simulink model "closedLoop_SpO2H"  (Simulink 10.0)
settings: Solver=ode23t  StartTime=0.0  StopTime=2000  FixedStep=0.01  RelTol=1e-6  AbsTol=1e-9
model workspace: external: MAT-File parL3.mat (data not in the file)
values from neighbouring files (symbols this model uses):
  a0 = parRp(3)    [calcAuxVars.m]    (also in parL.mat = [1.15338450687 1.39375935389 0.940877756773 0.999834385293 0; parL0.mat = [1.15338450687 1.39375935389 0.940877756773 0.999834385293 0; parL1.mat = [1.15338450687 1.39375935389 0.940877756773 0.999834385293 0; parL2.mat = [1.15338450687 1.39375935389 0.940877756773 0.999834385293 0)
  a1 = parRp(4)    [calcAuxVars.m]    (also in parL.mat = [0.343538892932 0.21152716103 0.0176956627984 0.500319126811; parL0.mat = [0.343538892932 0.21152716103 0.0176956627984 0.500319126811; parL1.mat = [0.343538892932 0.21152716103 0.0176956627984 0.500319126811; parL2.mat = [0.343538892932 0.21152716103 0.0176956627984 0.500319126811)
  a_p0 = 0.5    [parL.mat]    (also in parL0.mat; parL1.mat; parL2.mat; parL3.mat)
  b_p0 = 1.1    [parL.mat]    (also in parL0.mat; parL1.mat; parL2.mat; parL3.mat)
  c0 = parRp(5)    [calcAuxVars.m]    (also in parL.mat = [2.87886478699 3.35726152565 2.07888198195 3.00150379853 2.7; parL0.mat = [2.87886478699 3.35726152565 2.07888198195 3.00150379853 2.7; parL1.mat = [2.87886478699 3.35726152565 2.07888198195 3.00150379853 2.7; parL2.mat = [2.87886478699 3.35726152565 2.07888198195 3.00150379853 2.7)
  In_T = [4.28 3.84 4.92 31.48 4.84 4.16 4.04 6.28 22.04 4.52 4.2 4.2 ... (112 elements, 1x112)]    [parL.mat]    (also in parL0.mat; parL1.mat; parL2.mat; parL3.mat)
  InInspirT = [3.74988154254 3.29053790944 2.30955999915 3.3968770932 3.63249544085 3.4615806603 3.39373309529 2.87032279982 2.30291149597 3.50313332581 3.84662991695 3.66498954271 ... (112 elements, 112x1)]    [parL.mat]    (also in parL0.mat; parL1.mat; parL2.mat; parL3.mat)
  Ki = 0.0002    [parL.mat]    (also in parL0.mat; parL1.mat; parL2.mat = 0.002; parL3.mat = 0.002)
  Kp = 0.01    [parL.mat]    (also in parL0.mat = 0.04; parL1.mat = 0.04; parL2.mat = 0.4; parL3.mat = 0.4)
  LRI = 7.5    [parL.mat]    (also in parL0.mat; parL1.mat; parL2.mat = 6.5; parL3.mat = 6.5)
  Rp_adjust = 1    [parL.mat]    (also in parL0.mat; parL1.mat; parL2.mat; parL3.mat)
  SAo_set = 96    [parL2.mat]    (also in parL3.mat)
  taf = parRp(1)    [calcAuxVars.m]    (also in parL.mat = [0.808561437671 0.693291047527 0.236392042426 0.798691385589; parL0.mat = [0.808561437671 0.693291047527 0.236392042426 0.798691385589; parL1.mat = [0.808561437671 0.693291047527 0.236392042426 0.798691385589; parL2.mat = [0.808561437671 0.693291047527 0.236392042426 0.798691385589)
  tbf = parRp(2)+parRp(1)    [calcAuxVars.m]    (also in parL.mat = [1.94132010487 1.59724686191 1.07316795672 1.59818570761 1.9; parL0.mat = [1.94132010487 1.59724686191 1.07316795672 1.59818570761 1.9; parL1.mat = [1.94132010487 1.59724686191 1.07316795672 1.59818570761 1.9; parL2.mat = [1.94132010487 1.59724686191 1.07316795672 1.59818570761 1.9)
  x0 = xi(end,:)    [fitLung_slp60m1.m]    (also in fitLung_slp67xm.m; fitSpO2_slp60m1.m; fitSpO2_slp67xm.m; initialVariables.m = [x1;x2;x3;x4;x5;x6;x7;x8;x9;x10;x11;x12])
libraries: dspsigops x8, simulink x1
settings Model: Creator=ceic208  LastModifiedBy=wai484  SimulationMode=accelerator  PauseTimes=12.2274
settings Model: LogicAnalyzerGraphicalSettings=|
  | {
  |   "cursors" : {
  |     "activeCursor" : 0,
  |     "lockedCursors" : [
  | 
  |     ],
  |     "startingCursor" : 0,
  |     "times" : [
  |       0
  |     ]
  |   },
  |   "global" : {
  |   },
  |   "panels" : [
  |     {
  |       "height" : 100,
  |       "startingTrace" : 0,
  |       "traces" : [
  |         {
  |           "signalId" : "c403b30c-f251-48ef-8f45-5741095cfd99",
  |           "type" : "wave"
  |         },
  |         {
  |           "signalId" : "18fa4ba5-052e-4074-9df1-028c4f90615a",
  |           "type" : "wave"
  |         },
  |         {
  |           "signalId" : "c514b470-b808-4634-b1ae-82d406deb028",
  |           "type" : "wave"
  |         },
  |         {
  |           "signalId" : "1a470e6e-5724-4372-8d16-b9d493f2bf0a",
  |           "type" : "wave"
  |         }
  |       ],
  |       "yOffset" : 0
  |     }
  |   ],
  |   "timeAxis" : {
  |     "pixelsPerSecond" : 0.4395
  |   },
  |   "trigger" : {
  |     "enabled" : false,
  |     "mode" : "once",
  |     "samples" : 200,
  |     "signals" : {
  |     },
  |     "stages" : [
  |       {
  |         "conditions" : [
  | 
  |         ],
  |         "operator" : "AND"
  |       }
  |     ]
  |   }
  | }
settings DataIOCC: SignalLogging=off  DSMLogging=off
settings OptimizationCC: LifeSpan=auto
settings DebuggingCC: UnderspecifiedInitializationDetection=Simplified  MergeDetectMultiDrivingBlocksExec=error  SFUnexpectedBacktrackingDiag=error  SFNoUnconditionalDefaultTransitionDiag=error  SFExecutionAtInitializationDiag=warning
settings HardwareCC: ProdBitPerPointer=64  ProdBitPerSizeT=64  ProdBitPerPtrDiffT=64  ProdLargestAtomicFloat=Float  ProdIntDivRoundTo=Zero  ProdEndianess=LittleEndian  ProdWordSize=64  ProdHWDeviceType=Intel->x86-64 (Windows64)
settings ModelReferenceCC: PropagateSignalLabelsOutOfModel=on
settings GRTTargetCC: TargetLangStandard=C99 (ISO)  CombineOutputUpdateFcns=on  GRTInterface=off
settings ConfigComp: CovMetricSettings=dwe  CovSaveCumulativeToWorkspaceVar=off  CovSaveSingleToWorkspaceVar=off

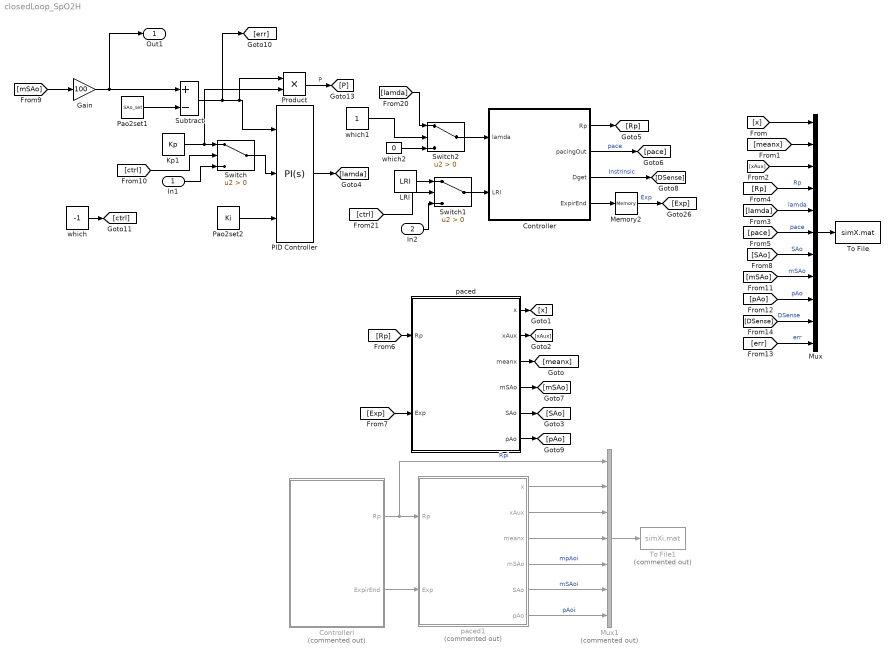
== system closedLoop_SpO2H ==
  In1 : Inport
  In2 : Inport  Port=2
  Controller : Stateflow chart  TreatAsAtomicUnit=on
  Controlleri : Stateflow chart  Commented=on  TreatAsAtomicUnit=on
  Gain : Gain  Gain=100
  Kp1 : Constant  Value=Kp  VectorParams1D=off
  LRI : Constant  Value=LRI  VectorParams1D=off
  Memory2 : Memory
  Mux : Mux  Inputs=11
  Mux1 : Mux  Commented=on  Inputs=7
  PID Controller : simulink/Continuous/PID Controller  Controller=PI  Form=Parallel  TimeDomain=Continuous-time  SampleTime=-1  IntegratorMethod=Forward Euler  FilterMethod=Forward Euler  ControllerParametersSource=external  P=Kp  I=Ki  D=0.00000000001  UseFilter=on  N=100  TunerSelectOption=Transfer Function Based (PID Tuner App)  InitialConditionSource=internal  InitialConditionForIntegrator=0  InitialConditionForFilter=0  DifferentiatorICPrevScaledInput=0  ExternalReset=none  TrackingMode=off  Kt=1  LimitOutput=on  UpperSaturationLimit=0.5  LowerSaturationLimit=-1.5  LinearizeAsGain=on  AntiWindupMode=none  Kb=1  POutMin=[]  POutMax=[]  IOutMin=[]  IOutMax=[]  DOutMin=[]  DOutMax=[]  NOutMin=[]  NOutMax=[]  SumOutMin=[]  SumOutMax=[]  SaturationOutMin=[]  SaturationOutMax=[]  PParamMin=[]  PParamMax=[]  IParamMin=[]  IParamMax=[]  DParamMin=[]  DParamMax=[]  NParamMin=[]  NParamMax=[]  KbParamMin=[]  KbParamMax=[]  KtParamMin=[]  KtParamMax=[]  KbOutMin=[]  KbOutMax=[]  KtOutMin=[]  KtOutMax=[]  IntegratorOutMin=[]  IntegratorOutMax=[]  FilterOutMin=[]  FilterOutMax=[]  SumI1OutMin=[]  SumI1OutMax=[]  SumI2OutMin=[]  SumI2OutMax=[]  SumI3OutMin=[]  SumI3OutMax=[]  SumI4OutMin=[]  SumI4OutMax=[]  SumDOutMin=[]  SumDOutMax=[]  DifferentiatorOutMin=[]  DifferentiatorOutMax=[]  FilterDiffOutCoefMin=[]  FilterDiffOutCoefMax=[]  ReciprocalOutMin=[]  ReciprocalOutMax=[]  SumDenOutMin=[]  SumDenOutMax=[]  SumNumOutMin=[]  SumNumOutMax=[]  DivideOutMin=[]  DivideOutMax=[]  IntegratorContinuousStateAttributes=''  IntegratorStateMustResolveToSignalObject=off  IntegratorRTWStateStorageClass=Auto  FilterContinuousStateAttributes=''  FilterStateMustResolveToSignalObject=off  FilterRTWStateStorageClass=Auto  ParallelPVariant=ExternalParameters  IdealPVariant=Disabled  IVariant=ExternalParameters  DVariant=Disabled  IntegratorVariant=Continuous  SatVariant=Enabled  AWVariant=Passthrough  PCopyVariant=Disabled  TRVariant=Disabled  FdbkBlocksVariant=Forward  IdealPFdbkVariant=Disabled  SatFdbkVariant=Disabled  DerivativeFilterVariant=Disabled  NVariant=Disabled  NCopyVariant=Disabled_SignalSpec  FilterICVariant=Disabled  IntegratorICVariant=InternalICs  ExternalResetVariant=Disabled  TRSumVariant=Passthrough  SumFdbkVariant=Disabled  SumVariant=Sum_PI
  Pao2set1 : Constant  Value=SAo_set  VectorParams1D=off
  Pao2set2 : Constant  Value=Ki  VectorParams1D=off
  Product : Product
  Subtract : Sum  Inputs=+-
  Switch : Switch  Criteria=u2 > Threshold
  Switch1 : Switch  Criteria=u2 > Threshold
  Switch2 : Switch  Criteria=u2 > Threshold
  To File : ToFile  Filename=simX.mat  MatrixName=simX
  To File1 : ToFile  Commented=on  Filename=simXi.mat  MatrixName=simXi
  paced : Subsystem
  paced1 : Subsystem  Commented=on
  which : Constant  Value=-1  VectorParams1D=off
  which1 : Constant  VectorParams1D=off
  which2 : Constant  Value=0  VectorParams1D=off
  Out1 : Outport  PortDimensions=1  VectorParamsAs1DForOutWhenUnconnected=off
  wires:
  Pao2set1/1 -> Subtract/2
  Subtract/1 -> [err], Product/1, PID Controller/1
  [x] -> Mux/1
  [meanx] -> Mux/2
  [xAux] -> Mux/3
  [Rp] -> Mux/4  "Rp"
  [lamda] -> Mux/5  "lamda"
  [pace] -> Mux/6  "pace"
  Mux/1 -> To File/1
  Controller/1(Rp) -> [Rp]
  Pao2set2/1 -> PID Controller/3
  PID Controller/1 -> [lamda]
  Controller/2(pacingOut) -> [pace]  "pace"
  Controller/3(Dget) -> [DSense]  "Instrinsic"
  Switch/1 -> PID Controller/2
  Kp1/1 -> Product/2, Switch/1
  In1/1 -> Switch/3
  which/1 -> [ctrl]
  [ctrl] -> Switch/2
  Switch1/1 -> Controller/2(LRI)
  LRI/1 -> Switch1/1
  In2/1 -> Switch1/3
  [ctrl] -> Switch1/2
  Memory2/1 -> [Exp]  "Exp"
  Controller/4(ExpirEnd) -> Memory2/1
  Product/1 -> [P]  "P"
  paced/3(meanx) -> [meanx]
  paced/1(x) -> [x]
  paced/2(xAux) -> [xAux]
  [Rp] -> paced/1(Rp)
  [Exp] -> paced/2(Exp)
  paced/5(SAo) -> [SAo]
  [SAo] -> Mux/7  "SAo"
  [mSAo] -> Mux/8  "mSAo"
  Controlleri/1(Rp) -> paced1/1(Rp), Mux1/1  "Rpi"
  Controlleri/2(ExpirEnd) -> paced1/2(Exp)
  Mux1/1 -> To File1/1
  paced1/1(x) -> Mux1/2
  paced/6(pAo) -> [pAo]
  paced1/2(xAux) -> Mux1/3
  paced1/3(meanx) -> Mux1/4
  paced1/4(mSAo) -> Mux1/5  "mpAoi"
  paced1/5(SAo) -> Mux1/6  "mSAoi"
  paced1/6(pAo) -> Mux1/7  "pAoi"
  [pAo] -> Mux/9  "pAo"
  [err] -> Mux/11  "err"
  [DSense] -> Mux/10  "DSense"
  [mSAo] -> Gain/1
  Gain/1 -> Out1/1, Subtract/1
  Switch2/1 -> Controller/1(lamda)
  [lamda] -> Switch2/1
  which1/1 -> Switch2/2
  which2/1 -> Switch2/3
  paced/4(mSAo) -> [mSAo]

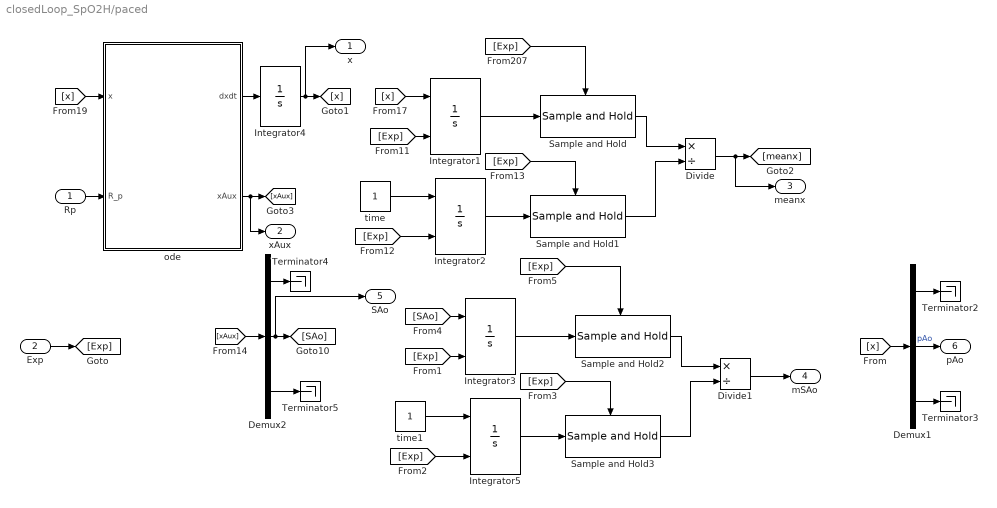
== system closedLoop_SpO2H/paced ==
  Rp : Inport
  Exp : Inport  Port=2
  Demux1 : Demux  Outputs=[6,1,5]
  Demux2 : Demux  Outputs=[13,1,1]
  Divide : Product  Inputs=*/
  Divide1 : Product  Inputs=*/
  Integrator{1..3,5} (4 alike) : Integrator  ExternalReset=either  LimitOutput=on  LowerSaturationLimit=0
  Integrator4 : Integrator  InitialCondition=x0  LimitOutput=on  LowerSaturationLimit=0
  Sample and Hold : dspsigops/Sample and Hold  trig=Either edge  initCond=x0  latchinput=on
  Sample and Hold1 : dspsigops/Sample and Hold  trig=Either edge  initCond=3  latchinput=on
  Sample and Hold2 : dspsigops/Sample and Hold  trig=Either edge  initCond=SAo_set/100*3  latchinput=on
  Sample and Hold3 : dspsigops/Sample and Hold  trig=Either edge  initCond=3  latchinput=on
  Terminator{2..5} (4 alike) : Terminator
  ode : MATLAB Function  TreatAsAtomicUnit=on
  time : Constant  VectorParams1D=off
  time1 : Constant  VectorParams1D=off
  x : Outport  VectorParamsAs1DForOutWhenUnconnected=off
  xAux : Outport  Port=2  VectorParamsAs1DForOutWhenUnconnected=off
  meanx : Outport  Port=3  VectorParamsAs1DForOutWhenUnconnected=off
  mSAo : Outport  Port=4  VectorParamsAs1DForOutWhenUnconnected=off
  SAo : Outport  Port=5  VectorParamsAs1DForOutWhenUnconnected=off
  pAo : Outport  Port=6  VectorParamsAs1DForOutWhenUnconnected=off
  wires:
  Divide/1 -> meanx/1, [meanx]
  time/1 -> Integrator2/1
  Demux2/2 -> SAo/1, [SAo]
  [Exp] -> Sample and Hold1/Trigger
  [Exp] -> Integrator2/2
  Sample and Hold/1 -> Divide/1
  Sample and Hold1/1 -> Divide/2
  [Exp] -> Integrator1/2
  Integrator4/1 -> x/1, [x]
  Integrator2/1 -> Sample and Hold1/1
  Integrator1/1 -> Sample and Hold/1
  [x] -> Integrator1/1
  [x] -> ode/1(x)
  ode/2(xAux) -> xAux/1, [xAux]
  ode/1(dxdt) -> Integrator4/1
  [xAux] -> Demux2/1
  Demux2/1 -> Terminator4/1
  [Exp] -> Sample and Hold/Trigger
  Demux2/3 -> Terminator5/1
  Rp/1 -> ode/2(R_p)
  Exp/1 -> [Exp]
  [x] -> Demux1/1
  Demux1/1 -> Terminator2/1
  Demux1/3 -> Terminator3/1
  Demux1/2 -> pAo/1  "pAo"
  [Exp] -> Sample and Hold2/Trigger
  Divide1/1 -> mSAo/1
  Sample and Hold2/1 -> Divide1/1
  Integrator5/1 -> Sample and Hold3/1
  Sample and Hold3/1 -> Divide1/2
  [Exp] -> Integrator5/2
  Integrator3/1 -> Sample and Hold2/1
  [SAo] -> Integrator3/1
  [Exp] -> Integrator3/2
  [Exp] -> Sample and Hold3/Trigger
  time1/1 -> Integrator5/1

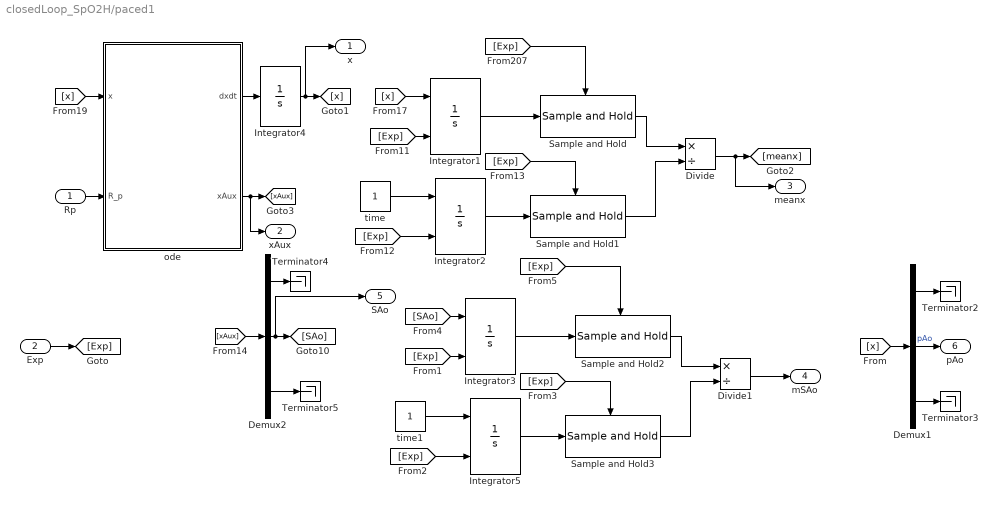
== system closedLoop_SpO2H/paced1 ==
  Rp : Inport
  Exp : Inport  Port=2
  Demux1 : Demux  Outputs=[6,1,5]
  Demux2 : Demux  Outputs=[13,1,1]
  Divide : Product  Inputs=*/
  Divide1 : Product  Inputs=*/
  Integrator{1..3,5} (4 alike) : Integrator  ExternalReset=either  LimitOutput=on  LowerSaturationLimit=0
  Integrator4 : Integrator  InitialCondition=x0  LimitOutput=on  LowerSaturationLimit=0
  Sample and Hold : dspsigops/Sample and Hold  trig=Either edge  initCond=x0  latchinput=on
  Sample and Hold1 : dspsigops/Sample and Hold  trig=Either edge  initCond=3  latchinput=on
  Sample and Hold2 : dspsigops/Sample and Hold  trig=Either edge  initCond=SAo_set/100*3  latchinput=on
  Sample and Hold3 : dspsigops/Sample and Hold  trig=Either edge  initCond=3  latchinput=on
  Terminator{2..5} (4 alike) : Terminator
  ode : MATLAB Function  TreatAsAtomicUnit=on
  time : Constant  VectorParams1D=off
  time1 : Constant  VectorParams1D=off
  x : Outport  VectorParamsAs1DForOutWhenUnconnected=off
  xAux : Outport  Port=2  VectorParamsAs1DForOutWhenUnconnected=off
  meanx : Outport  Port=3  VectorParamsAs1DForOutWhenUnconnected=off
  mSAo : Outport  Port=4  VectorParamsAs1DForOutWhenUnconnected=off
  SAo : Outport  Port=5  VectorParamsAs1DForOutWhenUnconnected=off
  pAo : Outport  Port=6  VectorParamsAs1DForOutWhenUnconnected=off
  wires:
  Divide/1 -> meanx/1, [meanx]
  time/1 -> Integrator2/1
  Demux2/2 -> SAo/1, [SAo]
  [Exp] -> Sample and Hold1/Trigger
  [Exp] -> Integrator2/2
  Sample and Hold/1 -> Divide/1
  Sample and Hold1/1 -> Divide/2
  [Exp] -> Integrator1/2
  Integrator4/1 -> x/1, [x]
  Integrator2/1 -> Sample and Hold1/1
  Integrator1/1 -> Sample and Hold/1
  [x] -> Integrator1/1
  [x] -> ode/1(x)
  ode/2(xAux) -> xAux/1, [xAux]
  ode/1(dxdt) -> Integrator4/1
  [xAux] -> Demux2/1
  Demux2/1 -> Terminator4/1
  [Exp] -> Sample and Hold/Trigger
  Demux2/3 -> Terminator5/1
  Rp/1 -> ode/2(R_p)
  Exp/1 -> [Exp]
  [x] -> Demux1/1
  Demux1/1 -> Terminator2/1
  Demux1/3 -> Terminator3/1
  Demux1/2 -> pAo/1  "pAo"
  [Exp] -> Sample and Hold2/Trigger
  Divide1/1 -> mSAo/1
  Sample and Hold2/1 -> Divide1/1
  Integrator5/1 -> Sample and Hold3/1
  Sample and Hold3/1 -> Divide1/2
  [Exp] -> Integrator5/2
  Integrator3/1 -> Sample and Hold2/1
  [SAo] -> Integrator3/1
  [Exp] -> Integrator3/2
  [Exp] -> Sample and Hold3/Trigger
  time1/1 -> Integrator5/1

== matlab function paced/ode ==
  data: dxdt output double; x input double; xAux output double; R_p input double; parL parameter double
% Calculates derivatives given x & t

function [dxdt,xAux] = odeSystem_LungSim(x,R_p, parL)

P_A = x(1);
f_o = x(2);
f_c = x(3);
f_do = x(4);
f_dc = x(5);
p_Vo = x(6);
p_Ao = x(7);
p_Vc = x(8);
p_Ac = x(9);
z_V = x(10);
z_A = x(11);
x_m=x(12);

[xAux] = calcAuxVarsSim(x,R_p, parL);

P_L = xAux(1);
dP_Ldt = xAux(2);
Q_A = xAux(3);
q = xAux(4);
p_ao = xAux(5);
p_ac = xAux(6);
V_A = xAux(7);
f_o_cos = xAux(8);
f_c_cos = xAux(9);
f_do_cos = xAux(10);
f_dc_cos = xAux(11);
dfpVodpVo = xAux(12);
dfpAodpAo = xAux(13);
S_Ao=xAux(14);
S_Vo=xAux(15);

p_bo = p_Ao; % p_b = partial pressure in pulmonary capillaries which does the flux
p_bc = p_Ac;

dx_mdt=-parL.k1.*x_m+parL.k2.*R_p;

dP_Adt = (parL.P_m.*parL.E.*Q_A)./P_A + dP_Ldt;

df_odt = (1./V_A).*((f_o_cos-f_o).*q + parL.Do.*(p_bo - p_ao) - f_o.*(parL.Dc.*(p_bc - p_ac) + parL.Do.*(p_bo - p_ao)));
df_cdt = (1./V_A).*((f_c_cos-f_c).*q + parL.Dc.*(p_bc - p_ac) - f_c.*(parL.Do.*(p_bo - p_ao) + parL.Dc.*(p_bc - p_ac)));

df_dodt = (1./parL.V_d).*(f_do_cos - f_do).*(abs(q));
df_dcdt = (1./parL.V_d).*(f_dc_cos - f_dc).*(abs(q));

% with blood flux from haemoglobin O2 binding
dp_Aodt = (1./parL.V_p).*((parL.sigma_o + 4.*parL.Th.*dfpAodpAo).^(-1)).*(parL.Dbo.*(p_ao - p_Ao) + parL.Q_CO.*parL.sigma_o.*(p_Vo - p_Ao) + parL.Q_CO.*4.*parL.Th.*(S_Vo - S_Ao));
dp_Vodt = (1./parL.V_s).*((parL.sigma_o + 4.*parL.Th.*dfpVodpVo).^(-1)).*(parL.M_o + parL.Q_CO.*parL.sigma_o.*(p_Ao - p_Vo) + parL.Q_CO.*4.*parL.Th.*(S_Ao - S_Vo));


dp_Acdt = (parL.Q_CO./parL.V_p).*(p_Vc - p_Ac) + (parL.Dbc./(parL.V_p.*parL.sigma_c)).*(p_ac - p_Ac) + (parL.delta.*parL.l2.*z_A.*parL.h)./(parL.sigma_c) - (parL.delta.*parL.r2.*p_Ac);
dp_Vcdt = (parL.Q_CO./parL.V_s).*(p_Ac - p_Vc) + (parL.M_c./(parL.V_s.*parL.sigma_c)) + (parL.delta.*parL.l2.*z_V.*parL.h)./(parL.sigma_c) - (parL.delta.*parL.r2.*p_Vc);

% with blood flux from bicarbonate
dz_Adt = (parL.delta.*parL.r2.*parL.sigma_c.*p_Ac) - (parL.delta.*parL.l2.*z_A.*parL.h) + (parL.Q_CO./parL.V_p).*(z_V - z_A);
dz_Vdt = (parL.delta.*parL.r2.*parL.sigma_c.*p_Vc) - (parL.delta.*parL.l2.*z_V.*parL.h) + (parL.Q_CO./parL.V_s).*(z_A - z_V);

dxdt = [dP_Adt; df_odt; df_cdt; df_dodt; df_dcdt; dp_Vodt; dp_Aodt; dp_Vcdt; dp_Acdt; dz_Vdt; dz_Adt;dx_mdt];
return
% Calculate auxiliary variables given x & t

function [xAux] = calcAuxVarsSim(x,R_p, parL)

P_A = x(1);
f_o = x(2);
f_c = x(3);
f_do = x(4);
f_dc = x(5);
p_Vo = x(6);
p_Ao = x(7);
p_Vc = x(8);
p_Ac = x(9);
z_V = x(10);
z_A = x(11);
x_m=x(12);

P_L=parL.P_m-parL.PL0-parL.kp.*x_m;
dP_Ldt=parL.k1.*parL.kp.*x_m-parL.k2.*parL.kp.*R_p;

p_bo = p_Ao; % p_b = partial pressure in pulmonary capillaries which does the flux
p_bc = p_Ac;

p_ao = f_o.*(P_A - parL.p_w);
p_ac = f_c.*(P_A - parL.p_w);

q = (parL.P_m - P_A)./parL.R;
Q_A = q + parL.Dc.*(p_bc - p_ac) + parL.Do.*(p_bo - p_ao);

V_A = (P_A - P_L)./parL.E + parL.V_0;

% f_o_cos & f_c_cos = transfer between alveoli and dead-space
% f_do_cos & f_dc_cos = transfer between dead-space and atmospheric gas

if(q > 0)     % inspiration (q)
    f_o_cos = f_do;
    f_c_cos = f_dc;
    f_do_cos = parL.f_mo;
    f_dc_cos = parL.f_mc;
elseif(q < 0) % expiration (q)
    f_o_cos = f_o;
    f_c_cos = f_c;
    f_do_cos = f_o;
    f_dc_cos = f_c;
else % q = 0 initially since P_A = P_m
    f_o_cos = f_o;
    f_c_cos = f_c;
    f_do_cos = f_o;
    f_dc_cos = f_c;
end

% O2-haemoglobin binding Monod-Wyman-Changeux
[dfpVodpVo] = calcSaturationGradient(p_Vo, parL);
[dfpAodpAo] = calcSaturationGradient(p_Ao, parL);

S_Ao = calcSaturation(p_Ao, parL);
S_Vo = calcSaturation(p_Vo, parL);

xAux = [P_L;dP_Ldt;Q_A;q;p_ao;p_ac;V_A;f_o_cos;f_c_cos;f_do_cos;f_dc_cos;dfpVodpVo;dfpAodpAo;S_Ao;S_Vo];
return
% Calculate O2-haemoglobin saturation function - Monod-Wyman-Changeux (MWC)

function [fpo] = calcSaturation(po, parL)

% A = L.*KT.*sigma_o.*po.*((1 + KT.*sigma_o.*po).^3);
% B = KR.*sigma_o.*po.*((1 + KR.*sigma_o.*po).^3);
% C = L.*(1 + KT.*sigma_o.*po).^4;
% D = (1 + KR.*sigma_o.*po).^4;
% fpo = (A + B)./(C + D);

A = parL.L.*parL.KT.*parL.sigma_o;
B = parL.KT.*parL.sigma_o;
C = parL.KR.*parL.sigma_o;

G = A.*po.*((1 + B.*po).^3) + C.*po.*((1 + C.*po).^3);
H = parL.L.*((1 + B.*po).^4) + (1 + C.*po).^4;
fpo = G./H;

return

% Calculate O2-haemoglobin binding curve gradient

% Check wolfram: differentiate y=((a*x*(1+b*x)^3) + (c*x*(1+ d*x)^3))/(e*(1+f*x)^4 + (1+ g*x)^4)

function [dfdpo] = calcSaturationGradient(po, parL)
% O2-haemoglobin binding
A = parL.L.*parL.KT.*parL.sigma_o;
B = parL.KT.*parL.sigma_o;
C = parL.KR.*parL.sigma_o;

G = A.*po.*((1 + B.*po).^3) + C.*po.*((1 + C.*po).^3);
H = parL.L.*((1 + B.*po).^4) + (1 + C.*po).^4;
Hsqrd = H.^2;
dGdpo = A.*((1 + B.*po).^2).*(1 + 4.*B.*po) + C.*((1 + C.*po).^2).*(1 + 4.*C.*po);
dHdpo = 4.*(parL.L.*B.*((1 + B.*po).^3) + C.*((1 + C.*po).^3));
dfdpo = ((dGdpo.*H) - (G.*dHdpo))./(Hsqrd);
return

== stateflow chart Controlleri ==
  state PNA % Phrenic Nerve Activity [parallel]
    entry: i=1; IT = In_T(i); InsT=0;InspirT = InInspirT(i);
    settings: executionOrder=1
    state ActiveIntrinsic % Inspiration
      entry: t0 = t;
      during: Rp = Rp_adjust*(a0(i)*(t-t0)./((t-t0)+a1(i)).*((t-t0)<=taf(i)) + ...
      ( ( a0(i).*a1(i)./(a1(i)+taf(i)).^2).*(t-t0)+(a0(i).*taf(i)./(taf(i)+a1(i)) ...
      -  ( a0(i).*a1(i)./(a1(i)+taf(i)).^2).*taf(i))) .* ((t-t0)<=tbf(i)&(t-t0)>taf(i)) + ...
      (( a0(i).*a1(i)./(a1(i)+taf(i)).^2)*tbf(i)+(a0(i).*taf(i)./(taf(i)+a1(i))...
      -  ( a0(i).*a1(i)./(a1(i)+taf(i)).^2).*taf(i)))*exp(-c0(i)*((t-t0)-tbf(i))).*((t-t0)>tbf(i)));
    state Inactive % Expiration
      entry: Rp = 0;
    (default) -> Inactive % Expiration
    Inactive % Expiration -> ActiveIntrinsic % Inspiration : [after(IT-InsT,sec)]
        | {send(ExpirEnd);}
    ActiveIntrinsic % Inspiration -> Inactive % Expiration : after(InspirT,sec)
        | {i=i+1;IT = In_T(i); InsT=InspirT;...
        | InspirT = InInspirT(i);}
  state wakeup [parallel]
    settings: executionOrder=2
    state per5s
    (default) -> per5s : {Rp=0;}
    per5s -> per5s : [Rp==0 &&after (5,sec)]
        | {send(ExpirEnd);}
  note: If breathing pauses, every 5 second, the PI controller sampes the blood gas;
  data: IT local double; Rp output double =0; t0 local double; InspirT local double; i local double; InInspirT parameter double; In_T parameter double; taf parameter double; tbf parameter double; a0 parameter double; a1 parameter double; c0 parameter double; Rp_adjust parameter double; InsT local double
  events: ExpirEnd output EITHER_EDGE_EVENT

== matlab function paced1/ode ==
  data: dxdt output double; x input double; xAux output double; R_p input double; parL parameter double
% Calculates derivatives given x & t

function [dxdt,xAux] = odeSystem_LungSim(x,R_p, parL)

P_A = x(1);
f_o = x(2);
f_c = x(3);
f_do = x(4);
f_dc = x(5);
p_Vo = x(6);
p_Ao = x(7);
p_Vc = x(8);
p_Ac = x(9);
z_V = x(10);
z_A = x(11);
x_m=x(12);

[xAux] = calcAuxVarsSim(x,R_p, parL);

P_L = xAux(1);
dP_Ldt = xAux(2);
Q_A = xAux(3);
q = xAux(4);
p_ao = xAux(5);
p_ac = xAux(6);
V_A = xAux(7);
f_o_cos = xAux(8);
f_c_cos = xAux(9);
f_do_cos = xAux(10);
f_dc_cos = xAux(11);
dfpVodpVo = xAux(12);
dfpAodpAo = xAux(13);
S_Ao=xAux(14);
S_Vo=xAux(15);

p_bo = p_Ao; % p_b = partial pressure in pulmonary capillaries which does the flux
p_bc = p_Ac;

dx_mdt=-parL.k1.*x_m+parL.k2.*R_p;

dP_Adt = (parL.P_m.*parL.E.*Q_A)./P_A + dP_Ldt;

df_odt = (1./V_A).*(f_o_cos.*q + parL.Do.*(p_bo - p_ao) - f_o.*(parL.Dc.*(p_bc - p_ac) + parL.Do.*(p_bo - p_ao)));
df_cdt = (1./V_A).*(f_c_cos.*q + parL.Dc.*(p_bc - p_ac) - f_c.*(parL.Do.*(p_bo - p_ao) + parL.Dc.*(p_bc - p_ac)));

df_dodt = (1./parL.V_d).*(f_do_cos - f_do).*(abs(q));
df_dcdt = (1./parL.V_d).*(f_dc_cos - f_dc).*(abs(q));

% with blood flux from haemoglobin O2 binding
dp_Aodt = (1./parL.V_p).*((parL.sigma_o + 4.*parL.Th.*dfpAodpAo).^(-1)).*(parL.Dbo.*(p_ao - p_Ao) + parL.Q_CO.*parL.sigma_o.*(p_Vo - p_Ao) + parL.Q_CO.*4.*parL.Th.*(S_Vo - S_Ao));
dp_Vodt = (1./parL.V_s).*((parL.sigma_o + 4.*parL.Th.*dfpVodpVo).^(-1)).*(parL.M_o + parL.Q_CO.*parL.sigma_o.*(p_Ao - p_Vo) + parL.Q_CO.*4.*parL.Th.*(S_Ao - S_Vo));


dp_Acdt = (parL.Q_CO./parL.V_p).*(p_Vc - p_Ac) + (parL.Dbc./(parL.V_p.*parL.sigma_c)).*(p_ac - p_Ac) + (parL.delta.*parL.l2.*z_A.*parL.h)./(parL.sigma_c) - (parL.delta.*parL.r2.*p_Ac);
dp_Vcdt = (parL.Q_CO./parL.V_s).*(p_Ac - p_Vc) + (parL.M_c./(parL.V_s.*parL.sigma_c)) + (parL.delta.*parL.l2.*z_V.*parL.h)./(parL.sigma_c) - (parL.delta.*parL.r2.*p_Vc);

% with blood flux from bicarbonate
dz_Adt = (parL.delta.*parL.r2.*parL.sigma_c.*p_Ac) - (parL.delta.*parL.l2.*z_A.*parL.h) + (parL.Q_CO./parL.V_p).*(z_V - z_A);
dz_Vdt = (parL.delta.*parL.r2.*parL.sigma_c.*p_Vc) - (parL.delta.*parL.l2.*z_V.*parL.h) + (parL.Q_CO./parL.V_s).*(z_A - z_V);

dxdt = [dP_Adt; df_odt; df_cdt; df_dodt; df_dcdt; dp_Vodt; dp_Aodt; dp_Vcdt; dp_Acdt; dz_Vdt; dz_Adt;dx_mdt];
return
% Calculate auxiliary variables given x & t

function [xAux] = calcAuxVarsSim(x,R_p, parL)

P_A = x(1);
f_o = x(2);
f_c = x(3);
f_do = x(4);
f_dc = x(5);
p_Vo = x(6);
p_Ao = x(7);
p_Vc = x(8);
p_Ac = x(9);
z_V = x(10);
z_A = x(11);
x_m=x(12);

P_L=parL.P_m-parL.PL0-parL.kp.*x_m;
dP_Ldt=parL.k1.*parL.kp.*x_m-parL.k2.*parL.kp.*R_p;

p_bo = p_Ao; % p_b = partial pressure in pulmonary capillaries which does the flux
p_bc = p_Ac;

p_ao = f_o.*(P_A - parL.p_w);
p_ac = f_c.*(P_A - parL.p_w);

q = (parL.P_m - P_A)./parL.R;
Q_A = q + parL.Dc.*(p_bc - p_ac) + parL.Do.*(p_bo - p_ao);

V_A = (P_A - P_L)./parL.E + parL.V_0;

% f_o_cos & f_c_cos = transfer between alveoli and dead-space
% f_do_cos & f_dc_cos = transfer between dead-space and atmospheric gas

if(q > 0)     % inspiration (q)
    f_o_cos = f_do;
    f_c_cos = f_dc;
    f_do_cos = parL.f_mo;
    f_dc_cos = parL.f_mc;
elseif(q < 0) % expiration (q)
    f_o_cos = f_o;
    f_c_cos = f_c;
    f_do_cos = f_o;
    f_dc_cos = f_c;
else % q = 0 initially since P_A = P_m
    f_o_cos = f_o;
    f_c_cos = f_c;
    f_do_cos = f_o;
    f_dc_cos = f_c;
end

% O2-haemoglobin binding Monod-Wyman-Changeux
[dfpVodpVo] = calcSaturationGradient(p_Vo, parL);
[dfpAodpAo] = calcSaturationGradient(p_Ao, parL);

S_Ao = calcSaturation(p_Ao, parL);
S_Vo = calcSaturation(p_Vo, parL);

xAux = [P_L;dP_Ldt;Q_A;q;p_ao;p_ac;V_A;f_o_cos;f_c_cos;f_do_cos;f_dc_cos;dfpVodpVo;dfpAodpAo;S_Ao;S_Vo];
return
% Calculate O2-haemoglobin saturation function - Monod-Wyman-Changeux (MWC)

function [fpo] = calcSaturation(po, parL)

% A = L.*KT.*sigma_o.*po.*((1 + KT.*sigma_o.*po).^3);
% B = KR.*sigma_o.*po.*((1 + KR.*sigma_o.*po).^3);
% C = L.*(1 + KT.*sigma_o.*po).^4;
% D = (1 + KR.*sigma_o.*po).^4;
% fpo = (A + B)./(C + D);

A = parL.L.*parL.KT.*parL.sigma_o;
B = parL.KT.*parL.sigma_o;
C = parL.KR.*parL.sigma_o;

G = A.*po.*((1 + B.*po).^3) + C.*po.*((1 + C.*po).^3);
H = parL.L.*((1 + B.*po).^4) + (1 + C.*po).^4;
fpo = G./H;

return

% Calculate O2-haemoglobin binding curve gradient

% Check wolfram: differentiate y=((a*x*(1+b*x)^3) + (c*x*(1+ d*x)^3))/(e*(1+f*x)^4 + (1+ g*x)^4)

function [dfdpo] = calcSaturationGradient(po, parL)
% O2-haemoglobin binding
A = parL.L.*parL.KT.*parL.sigma_o;
B = parL.KT.*parL.sigma_o;
C = parL.KR.*parL.sigma_o;

G = A.*po.*((1 + B.*po).^3) + C.*po.*((1 + C.*po).^3);
H = parL.L.*((1 + B.*po).^4) + (1 + C.*po).^4;
Hsqrd = H.^2;
dGdpo = A.*((1 + B.*po).^2).*(1 + 4.*B.*po) + C.*((1 + C.*po).^2).*(1 + 4.*C.*po);
dHdpo = 4.*(parL.L.*B.*((1 + B.*po).^3) + C.*((1 + C.*po).^3));
dfdpo = ((dGdpo.*H) - (G.*dHdpo))./(Hsqrd);
return

== stateflow chart Controller ==
  state PacingController [parallel]
    settings: executionOrder=1
    state LRI_timer
    (default) -> LRI_timer
    LRI_timer -> LRI_timer [order 1] : DSense
    LRI_timer -> LRI_timer [order 2] : [after(LRI,sec)]{send(DPace,PNA);...
        | send(DPace,Sensing);send(ExpirEnd);}
  state Sensing [parallel]
    settings: executionOrder=3
    state active
    state Inactive
    (default) -> Inactive : {Dget=0;}
    Inactive -> active [order 1] : DPace
    Inactive -> active [order 2] : [Rp>0.65 && pacingOut==0]
        | {send(DSense,PacingController);...
        | send(ExpirEnd);Dget=1;}
    active -> Inactive : [Rp<0.1]{Dget=0;}
  state PNA % Phrenic Nerve Activity [parallel]
    entry: i=1; IT = In_T(i); InsT=0;InspirT = InInspirT(i);InspirT_p=LRI./3;
    settings: executionOrder=2
    state ActiveIntrinsic % Inspiration
      entry: t0 = t;
      during: Rp = Rp_adjust*(a0(i)*(t-t0)./((t-t0)+a1(i)).*((t-t0)<=taf(i)) + ...
      ( ( a0(i).*a1(i)./(a1(i)+taf(i)).^2).*(t-t0)+(a0(i).*taf(i)./(taf(i)+a1(i)) ...
      -  ( a0(i).*a1(i)./(a1(i)+taf(i)).^2).*taf(i))) .* ((t-t0)<=tbf(i)&(t-t0)>taf(i)) + ...
      (( a0(i).*a1(i)./(a1(i)+taf(i)).^2)*tbf(i)+(a0(i).*taf(i)./(taf(i)+a1(i))...
      -  ( a0(i).*a1(i)./(a1(i)+taf(i)).^2).*taf(i)))*exp(-c0(i)*((t-t0)-tbf(i))).*((t-t0)>tbf(i)));
    state Inactive % Expiration
      entry: Rp = 0;
      entry: pacingOut = 0;
    state del
    state ActivePacing % Inspiration
      entry: t0 = t; InsT=0; pacingOut = 1;
      a_p =(1-lamda)*a_p0;
      b_p =(1-lamda)*b_p0;
      during: Rp =  a_p+(b_p-a_p)/InspirT_p*(t-t0);
    (default) -> Inactive % Expiration
    Inactive % Expiration -> Inactive % Expiration [order 1] : [IT-InsT<=0.5]{i=i+1;IT = In_T(i);InspirT = InInspirT(i);}
    Inactive % Expiration -> ActiveIntrinsic % Inspiration [order 2] : [IT-InsT>0.5 && after(IT-InsT,sec)]
    ActiveIntrinsic % Inspiration -> Inactive % Expiration [order 1] : after(InspirT,sec)
        | {i=i+1;IT = In_T(i); InsT=InspirT;...
        | InspirT = InInspirT(i);}
    ActivePacing % Inspiration -> Inactive % Expiration : after(InspirT_p,sec)
        | {InsT=InspirT_p;}
    Inactive % Expiration -> del [order 3] : DPace{IT=IT-LRI;}
    ActiveIntrinsic % Inspiration -> del [order 2] : DPace{i=i+1;IT = In_T(i); InspirT = InInspirT(i);}
    del -> ActivePacing % Inspiration : after(0.001,sec)
  data: IT local double; Rp output double =0; t0 local double; InspirT local double; i local double; InInspirT parameter double; In_T parameter double; taf parameter double; tbf parameter double; a0 parameter double; a1 parameter double; c0 parameter double; pacingOut output double; a_p0 parameter double; b_p0 parameter double; b_p local double =b_p0; a_p local double =a_p0; InspirT_p local double; Rp_adjust parameter double; InsT local double; lamda input double; LRI input double; Dget output double
  events: DPace local FUNCTION_CALL_EVENT; ExpirEnd output EITHER_EDGE_EVENT; DSense local EITHER_EDGE_EVENT
